simulink model "qpsk_system_2"  (Simulink 6.6)
settings: Solver=ode45  StartTime=0.0  StopTime=0.1  RelTol=1e-3
PreLoadFcn:
  | rrc_weights
  | filter_weights
StopFcn:
  | figure(10)
  | 
  | subplot(1,2,1)
  | hold off
  | plot(i_in(20:end),q_in(20:end),'bo','MarkerFaceColor','b','MarkerSize',4);
  | hold on
  | plot([0 0],[-1.2 1.2],'k:');
  | plot([-1.2 1.2], [0 0],'k:');
  | title('Constellation (Input)');
  | xlabel('In Phase');
  | ylabel('Quadrature');
  | axis([-1.2 1.2 -1.2 1.2]);
  | axis square;
  | 
  | subplot(1,2,2)
  | hold off
  | plot(i_out(20:end),q_out(20:end),'bo','MarkerFaceColor','b','MarkerSize',4);
  | hold on
  | plot([0 0],[-1.2 1.2],'k:');
  | plot([-1.2 1.2], [0 0],'k:');
  | title('Constellation (Output)');
  | xlabel('In Phase');
  | ylabel('Quadrature');
  | axis([-1.2 1.2 -1.2 1.2]);
  | axis square;
libraries: dspsigops x4, dsparch4 x4, simulink x2
settings Model: Creator=lcrockett  LastModifiedBy=lcrockett

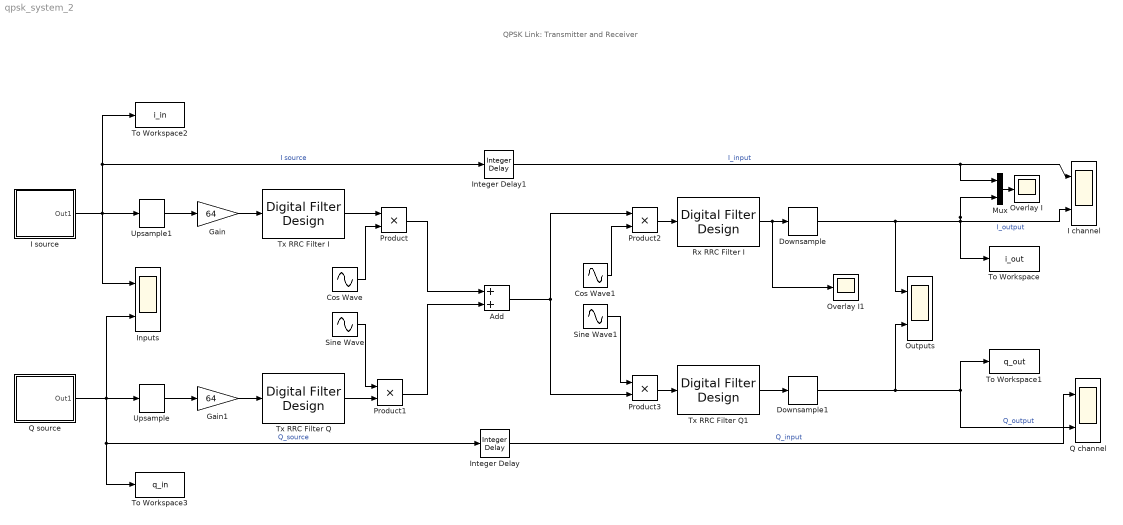
== system qpsk_system_2 ==
  note: QPSK Link: Transmitter and Receiver
  Add : Sum  OutScaling=2^-10
  Cos Wave : Sin  Frequency=(38.4e+3)*2*pi  Phase=pi/2  SampleTime=1/153.6e+3
  Cos Wave1 : Sin  Frequency=(38.4e+3)*2*pi  Phase=pi/2  SampleTime=1/153.6e+3
  Downsample : dspsigops/Downsample  N=64  phase=0  ic=0  smode=Allow multirate  fmode=Maintain input frame size
  Downsample1 : dspsigops/Downsample  N=64  phase=0  ic=0  smode=Allow multirate  fmode=Maintain input frame size
  Gain : Gain  Gain=64
  Gain1 : Gain  Gain=64
  I channel : Scope  NumInputPorts=2
      settings: YMin=-1.2~-1.2  YMax=1.2~1.2  SaveName=ScopeData2
  I source : Subsystem
  Inputs : Scope  NumInputPorts=2
      settings: YMin=-1.2~-1.2  YMax=1.2~1.2
  Integer Delay : simulink/Discrete/Integer Delay  vinit=0.0  samptime=-1  NumDelays=11
  Integer Delay1 : simulink/Discrete/Integer Delay  vinit=0  samptime=-1  NumDelays=11
  Mux : Mux  Inputs=2
  Outputs : Scope  NumInputPorts=2
      settings: YMin=-0.6~-0.6  YMax=0.6~0.6
  Overlay I : Scope
      settings: YMin=-1.5  YMax=1.5  SaveName=ScopeData4
  Overlay I1 : Scope
      settings: YMin=-1.5  YMax=1.5  SaveName=ScopeData5
  Product{,1..3} (4 alike) : Product  RndMeth=Zero
  Q channel : Scope  NumInputPorts=2
      settings: YMin=-1.2~-1.2  YMax=1.2~1.2  SaveName=ScopeData3
  Q source : Subsystem
  Rx RRC Filter I : dsparch4/Digital Filter Design  SystemSampleTime=-1  mwdsp_browser_bugfix_var=off
  Sine Wave : Sin  Frequency=(38.4e+3)*2*pi  SampleTime=1/153.6e+3
  Sine Wave1 : Sin  Frequency=(38.4e+3)*2*pi  SampleTime=1/153.6e+3
  To Workspace : ToWorkspace  VariableName=i_out  SampleTime=-1  SaveFormat=Array
  To Workspace1 : ToWorkspace  VariableName=q_out  SampleTime=-1  SaveFormat=Array
  To Workspace2 : ToWorkspace  VariableName=i_in  SampleTime=-1  SaveFormat=Array
  To Workspace3 : ToWorkspace  VariableName=q_in  SampleTime=-1  SaveFormat=Array
  Tx RRC Filter I : dsparch4/Digital Filter Design  SystemSampleTime=-1  mwdsp_browser_bugfix_var=off
  Tx RRC Filter Q : dsparch4/Digital Filter Design  SystemSampleTime=-1  mwdsp_browser_bugfix_var=off
  Tx RRC Filter Q1 : dsparch4/Digital Filter Design  SystemSampleTime=-1  mwdsp_browser_bugfix_var=off
  Upsample : dspsigops/Upsample  N=64  phase=0  ic=0  mode=Maintain input frame size
  Upsample1 : dspsigops/Upsample  N=64  phase=0  ic=0  mode=Maintain input frame size
  wires:
  Q source/1(Out1) -> Upsample/1, Inputs/2, Integer Delay/1, To Workspace3/1  "Q_source"
  Tx RRC Filter I/1 -> Product/1
  Tx RRC Filter Q/1 -> Product1/2
  Product/1 -> Add/1
  Product1/1 -> Add/2
  Add/1 -> Product2/1, Product3/2
  Upsample/1 -> Gain1/1
  I source/1(Out1) -> Upsample1/1, Inputs/1, Integer Delay1/1, To Workspace2/1  "I source"
  Upsample1/1 -> Gain/1
  Product2/1 -> Rx RRC Filter I/1
  Product3/1 -> Tx RRC Filter Q1/1
  Rx RRC Filter I/1 -> Downsample/1, Overlay I1/1
  Tx RRC Filter Q1/1 -> Downsample1/1
  Downsample/1 -> Outputs/1, I channel/2, Mux/2, To Workspace/1  "I_output"
  Downsample1/1 -> Outputs/2, Q channel/2, To Workspace1/1  "Q_output"
  Sine Wave/1 -> Product1/1
  Cos Wave/1 -> Product/2
  Sine Wave1/1 -> Product3/1
  Cos Wave1/1 -> Product2/2
  Integer Delay/1 -> Q channel/1  "Q_input"
  Integer Delay1/1 -> I channel/1, Mux/1  "I_input"
  Mux/1 -> Overlay I/1
  Gain/1 -> Tx RRC Filter I/1
  Gain1/1 -> Tx RRC Filter Q/1

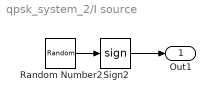
== system qpsk_system_2/I source ==
  Random Number2 : RandomNumber  Seed=777  SampleTime=1/2400
  Sign2 : Signum
  Out1 : Outport
  wires:
  Random Number2/1 -> Sign2/1
  Sign2/1 -> Out1/1

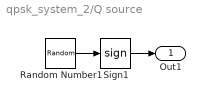
== system qpsk_system_2/Q source ==
  Random Number1 : RandomNumber  Seed=99  SampleTime=1/2400
  Sign1 : Signum
  Out1 : Outport
  wires:
  Random Number1/1 -> Sign1/1
  Sign1/1 -> Out1/1
